simulink model "arduino_smart_plant"  (R2024b)
settings: Solver=FixedStepAuto  StartTime=0.0  StopTime=100  RelTol=1e-3  EnableMultiTasking=on
undefined symbols (not defined in the file): Fi, Wi
libraries: arduinolib x4, arduinowifilib x4
settings Model: ExtModeTrigDuration=2  Creator=The MathWorks, Inc.  LastModifiedBy=ARJUN HUGAR
settings SolverCC: AlgebraicLoopSolver=TrustRegion
settings DataIOCC: ReturnWorkspaceOutputs=off
settings OptimizationCC: MaxStackSize=64
settings DebuggingCC: ParameterTunabilityLossMsg=error  UnconnectedInputMsg=warning  UnconnectedOutputMsg=warning  UnconnectedLineMsg=warning  ArithmeticOperatorsInVariantConditions=warning
settings HardwareCC: ProdBitPerInt=16  ProdBitPerPointer=16  ProdBitPerSizeT=16  ProdBitPerPtrDiffT=16  ProdLargestAtomicFloat=None  ProdWordSize=8  ProdHWDeviceType=Atmel->AVR  UseEmbeddedCoderFeatures=off  UseSimulinkCoderFeatures=off
settings ModelReferenceCC: EnableRefExpFcnMdlSchedulingChecks=on
settings SFSimCC: SimUseLocalCustomCode=off
settings RTWCC: Description=Embedded Coder  SystemTargetFile=ert.tlc  HardwareBoard=Arduino Mega 2560  TemplateMakefile=ert_default_tmf  GenerateReport=on  RTWUseLocalCustomCode=off  Toolchain=Arduino AVR  BuildConfiguration=Faster Runs  LaunchReport=on  GPUComputeCapability=3.5
settings CodeAppCC: ForceParamTrailComments=on  OperatorAnnotations=on  StateflowObjectComments=on  MATLABSourceComments=on
settings ERTTargetCC: ERTCustomFileBanners=off  SupportContinuousTime=on  SupportNonInlinedSFcns=on  RemoveResetFunc=off  SupportVariableSizeSignals=on  ModelStepFunctionPrototypeControlCompliant=off  InlinedParameterPlacement=Hierarchical  DynamicArrayContainerType=coder::array

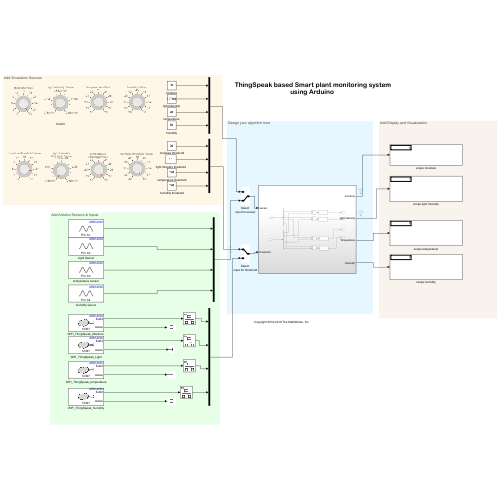
[thumbnail: Simulink's stored preview of the top-level diagram]
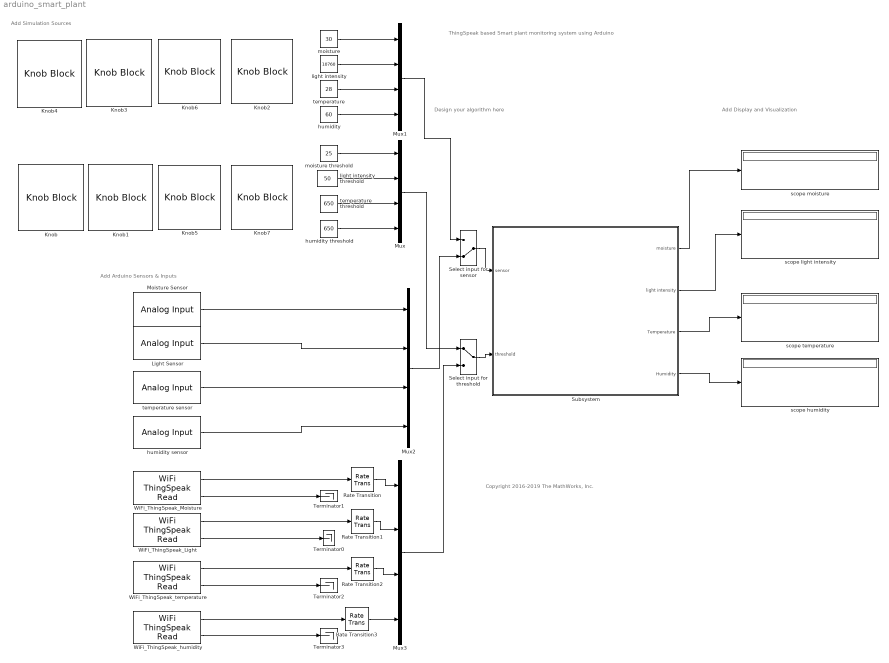
== system arduino_smart_plant ==
  note: Add Display and Visualization
  note: ThingSpeak based Smart plant monitoring system
      | using Arduino
  note: Add Simulation Sources
  note: Design your algorithm here
  note: Add Arduino Sensors & Inputs
  note: Copyright 2016-2019 The MathWorks, Inc.
  " humidity threshold" : Constant  Value=650  OutDataTypeStr=uint16
  " moisture threshold" : Constant  Value=25  OutDataTypeStr=uint16
  " temperature threshold" : Constant  Value=650  OutDataTypeStr=uint16
  Knob : KnobBlock  ScaleMax=30
  Knob1 : KnobBlock  ScaleMin=10760  ScaleMax=26900
  Knob2 : KnobBlock  ScaleMin=30  ScaleMax=60
  Knob3 : KnobBlock  ScaleMin=10760  ScaleMax=26900
  Knob4 : KnobBlock  ScaleMax=30
  Knob5 : KnobBlock  ScaleMin=18  ScaleMax=28
  Knob6 : KnobBlock  ScaleMin=18  ScaleMax=28
  Knob7 : KnobBlock  ScaleMin=30  ScaleMax=60
  Light Sensor : arduinolib/Analog Input  pinNumber=0  ReadResultsOnly=off  ConversionTriggerSource=Software  ExternalTriggerType=uint32(0)  OutputDataType=uint16  EnableConversionCompleteNotify=off  EnableOuputStatus=off  SampleTime=2  blockPlatform=arduino
      settings: SourceProductName=Common
  Moisture Sensor : arduinolib/Analog Input  pinNumber=1  ReadResultsOnly=off  ConversionTriggerSource=Software  ExternalTriggerType=uint32(0)  OutputDataType=uint16  EnableConversionCompleteNotify=off  EnableOuputStatus=off  SampleTime=2  blockPlatform=arduino
      settings: SourceProductName=Common
  Mux{,1..3} (4 alike) : Mux
  Rate Transition{,1..3} (4 alike) : RateTransition  OutPortSampleTime=2
  Select input for sensor : ManualSwitch  CurrentSetting=0
  Select input for threshold : ManualSwitch
  Subsystem : Subsystem
  Terminator{0..3} (4 alike) : Terminator
  WiFi_ThingSpeak_Light : arduinowifilib/WiFi ThingSpeak Read  ChannelID_=12397  Interfacetype_=Wi-Fi  ChannelAccess_=Public  ReadAPIKey_=ABCDEFGHIJK  FieldsToRead_=3  PrintDiagnosticMessages_=off  SampleTime_=60  blockPlatform=Arduino
  "WiFi_ThingSpeak_Moisture " : arduinowifilib/WiFi ThingSpeak Read  ChannelID_=12397  Interfacetype_=Wi-Fi  ChannelAccess_=Public  ReadAPIKey_=ABCDEFGHIJK  FieldsToRead_=4  PrintDiagnosticMessages_=off  SampleTime_=60  blockPlatform=Arduino
  WiFi_ThingSpeak_humidity : arduinowifilib/WiFi ThingSpeak Read  ChannelID_=12397  Interfacetype_=Wi-Fi  ChannelAccess_=Public  ReadAPIKey_=ABCDEFGHIJK  FieldsToRead_=4  PrintDiagnosticMessages_=off  SampleTime_=60  blockPlatform=Arduino
  WiFi_ThingSpeak_temperature : arduinowifilib/WiFi ThingSpeak Read  ChannelID_=12397  Interfacetype_=Wi-Fi  ChannelAccess_=Public  ReadAPIKey_=ABCDEFGHIJK  FieldsToRead_=4  PrintDiagnosticMessages_=off  SampleTime_=60  blockPlatform=Arduino
  humidity : Constant  Value=60  OutDataTypeStr=uint16
  humidity sensor : arduinolib/Analog Input  pinNumber=4  ReadResultsOnly=off  ConversionTriggerSource=Software  ExternalTriggerType=uint32( 0 )  OutputDataType=uint16  EnableConversionCompleteNotify=off  EnableOuputStatus=off  SampleTime=-1  blockPlatform=arduino
      settings: SourceProductName=Common
  "light intensity " : Constant  Value=10760  OutDataTypeStr=uint16
  light intensity threshold : Constant  Value=50  OutDataTypeStr=uint16
  moisture : Constant  Value=30  OutDataTypeStr=uint16
  scope humidity : Display
  scope light intensity : Display
  scope moisture : Display
  scope temperature : Display
  temperature : Constant  Value=28  OutDataTypeStr=uint16
  temperature sensor : arduinolib/Analog Input  pinNumber=3  ReadResultsOnly=off  ConversionTriggerSource=Software  ExternalTriggerType=uint32( 0 )  OutputDataType=uint16  EnableConversionCompleteNotify=off  EnableOuputStatus=off  SampleTime=-1  blockPlatform=arduino
      settings: SourceProductName=Common
  wires:
  "light intensity "/1 -> Mux1/2
  Rate Transition/1 -> Mux3/1
  Subsystem/2(light intensity) -> scope light intensity/1
  WiFi_ThingSpeak_Light/2 -> Terminator0/1
  Subsystem/1(moisture) -> scope moisture/1
  Select input for sensor/1 -> Subsystem/1(sensor)
  "WiFi_ThingSpeak_Moisture "/1 -> Rate Transition/1
  Select input for threshold/1 -> Subsystem/2(threshold)
  Rate Transition1/1 -> Mux3/2
  light intensity threshold/1 -> Mux/2
  " moisture threshold"/1 -> Mux/1
  moisture/1 -> Mux1/1
  Moisture Sensor/1 -> Mux2/1
  Light Sensor/1 -> Mux2/2
  Mux1/1 -> Select input for sensor/1
  Mux2/1 -> Select input for sensor/2
  "WiFi_ThingSpeak_Moisture "/2 -> Terminator1/1
  Mux3/1 -> Select input for threshold/2
  WiFi_ThingSpeak_Light/1 -> Rate Transition1/1
  Mux/1 -> Select input for threshold/1
  temperature/1 -> Mux1/3
  humidity/1 -> Mux1/4
  " temperature threshold"/1 -> Mux/3
  " humidity threshold"/1 -> Mux/4
  temperature sensor/1 -> Mux2/3
  humidity sensor/1 -> Mux2/4
  WiFi_ThingSpeak_temperature/2 -> Terminator2/1
  WiFi_ThingSpeak_temperature/1 -> Rate Transition2/1
  Rate Transition2/1 -> Mux3/3
  Rate Transition3/1 -> Mux3/4
  WiFi_ThingSpeak_humidity/1 -> Rate Transition3/1
  WiFi_ThingSpeak_humidity/2 -> Terminator3/1
  Subsystem/3(Temperature) -> scope temperature/1
  Subsystem/4(Humidity) -> scope humidity/1

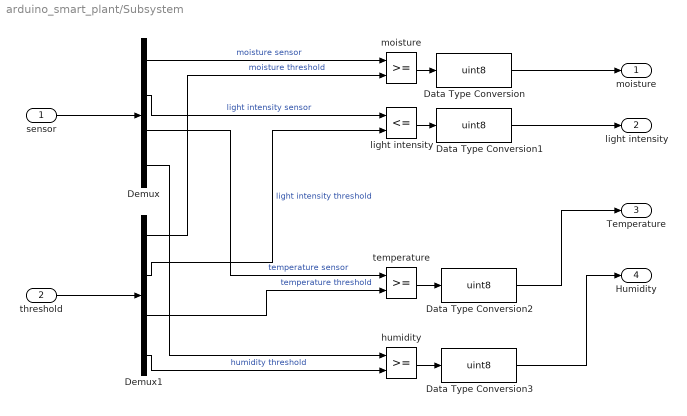
== system arduino_smart_plant/Subsystem ==
  sensor : Inport
  threshold : Inport  Port=2
  Data Type Conversion{,1..3} (4 alike) : DataTypeConversion  OutDataTypeStr=uint8  SaturateOnIntegerOverflow=off  RndMeth=Floor
  Demux : Demux
  Demux1 : Demux
  humidity : RelationalOperator  OutDataTypeStr=boolean  RndMeth=Simplest  InputSameDT=off
  "light intensity " : RelationalOperator  Operator=<=  OutDataTypeStr=boolean  RndMeth=Simplest  InputSameDT=off
  "moisture " : RelationalOperator  OutDataTypeStr=boolean  RndMeth=Simplest  InputSameDT=off
  temperature : RelationalOperator  OutDataTypeStr=boolean  RndMeth=Simplest  InputSameDT=off
  moisture : Outport  VectorParamsAs1DForOutWhenUnconnected=off
  light intensity : Outport  Port=2  VectorParamsAs1DForOutWhenUnconnected=off
  Temperature : Outport  Port=3  VectorParamsAs1DForOutWhenUnconnected=off
  Humidity : Outport  Port=4  VectorParamsAs1DForOutWhenUnconnected=off
  wires:
  sensor/1 -> Demux/1
  threshold/1 -> Demux1/1
  Demux/1 -> "moisture "/1  "moisture sensor"
  Demux1/1 -> "moisture "/2  "moisture threshold"
  Demux/2 -> "light intensity "/1  "light intensity sensor"
  Demux1/2 -> "light intensity "/2  "light intensity threshold"
  "moisture "/1 -> Data Type Conversion/1
  Data Type Conversion/1 -> moisture/1
  "light intensity "/1 -> Data Type Conversion1/1
  Data Type Conversion1/1 -> light intensity/1
  Demux/3 -> temperature/1  "temperature sensor"
  Demux1/3 -> temperature/2  "temperature threshold"
  temperature/1 -> Data Type Conversion2/1
  Data Type Conversion2/1 -> Temperature/1
  Demux1/4 -> humidity/2  "humidity threshold"
  humidity/1 -> Data Type Conversion3/1
  Data Type Conversion3/1 -> Humidity/1
  Demux/4 -> humidity/1
